simulink model "QuadrangleSimulation"  (R2022b)
settings: Solver=ode4  StartTime=0.0  StopTime=15  FixedStep=ts  MaxStep=0.6  RelTol=1e-3
values from neighbouring files (symbols this model uses):
  N = 20    [QuadrangleMain.m]
  p_left = []    [QuadrangleMain.m]
  p_right = []    [QuadrangleMain.m]
  ra = 0.8    [QuadrangleMain.m]
  rs = 0.5    [QuadrangleMain.m]
  vmax = 3    [QuadrangleMain.m]
settings Model: Creator=51078  LastModifiedBy=51078
settings SolverCC: AlgebraicLoopSolver=TrustRegion
settings DataIOCC: ReturnWorkspaceOutputs=off
settings DebuggingCC: UnconnectedInputMsg=warning  UnconnectedOutputMsg=warning  UnconnectedLineMsg=warning  SFMachineParentedDataDiag=warning  ArithmeticOperatorsInVariantConditions=warning
settings ModelReferenceCC: EnableRefExpFcnMdlSchedulingChecks=on
settings SFSimCC: SimUseLocalCustomCode=off  CustomCodeUndefinedFunction=UseInterfaceOnly
settings RTWCC: RTWUseLocalCustomCode=off  DLArmComputeVersion=19.05
settings CodeAppCC: StateflowObjectComments=on

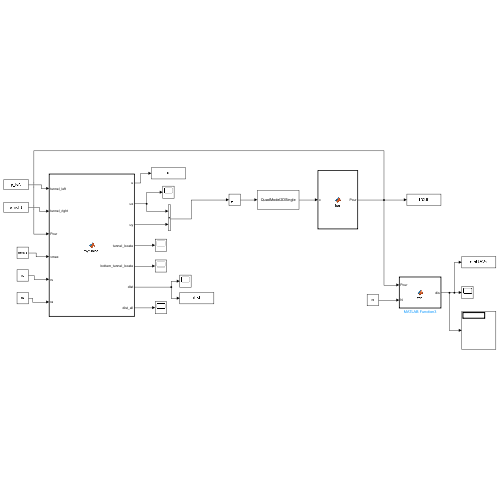
[thumbnail: Simulink's stored preview of the top-level diagram]
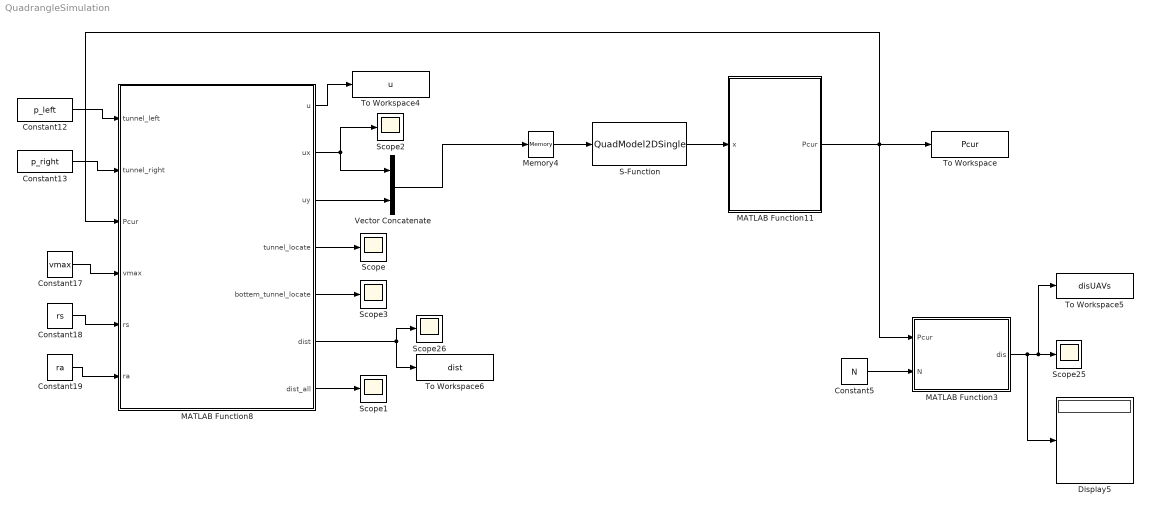
== system QuadrangleSimulation ==
  Constant12 : Constant  Value=p_left
  Constant13 : Constant  Value=p_right
  Constant17 : Constant  Value=vmax
  Constant18 : Constant  Value=rs
  Constant19 : Constant  Value=ra
  Constant5 : Constant  Value=N
  Display5 : Display
  MATLAB Function11 : MATLAB Function  TreatAsAtomicUnit=on
  MATLAB Function3 : MATLAB Function  TreatAsAtomicUnit=on
  MATLAB Function8 : MATLAB Function  TreatAsAtomicUnit=on
  Memory4 : Memory
  S-Function : S-Function  FunctionName=QuadModel2DSingle  SFunctionDeploymentMode=off  EnableBusSupport=off
  Scope{,1..3,25..26} (6 alike) : Scope
  To Workspace : ToWorkspace  VariableName=Pcur  SaveFormat=Timeseries  SampleTime=-1
  To Workspace4 : ToWorkspace  VariableName=u  SaveFormat=Timeseries  SampleTime=-1
  To Workspace5 : ToWorkspace  VariableName=disUAVs  SaveFormat=Timeseries  SampleTime=-1
  To Workspace6 : ToWorkspace  VariableName=dist  SaveFormat=Timeseries  SampleTime=-1
  Vector Concatenate : Concatenate
  wires:
  MATLAB Function8/4(tunnel_locate) -> Scope/1
  Constant12/1 -> MATLAB Function8/1(tunnel_left)
  Constant13/1 -> MATLAB Function8/2(tunnel_right)
  Constant17/1 -> MATLAB Function8/4(vmax)
  Constant18/1 -> MATLAB Function8/5(rs)
  Constant19/1 -> MATLAB Function8/6(ra)
  MATLAB Function11/1(Pcur) -> MATLAB Function8/3(Pcur), To Workspace/1, MATLAB Function3/1(Pcur)
  MATLAB Function3/1(dis) -> Display5/1, To Workspace5/1, Scope25/1
  Constant5/1 -> MATLAB Function3/2(N)
  MATLAB Function8/6(dist) -> Scope26/1, To Workspace6/1
  Memory4/1 -> S-Function/1
  MATLAB Function8/1(u) -> To Workspace4/1
  S-Function/1 -> MATLAB Function11/1(x)
  MATLAB Function8/3(uy) -> Vector Concatenate/2
  MATLAB Function8/2(ux) -> Scope2/1, Vector Concatenate/1
  Vector Concatenate/1 -> Memory4/1
  MATLAB Function8/5(bottem_tunnel_locate) -> Scope3/1
  MATLAB Function8/7(dist_all) -> Scope1/1

== matlab function QuadrangleSimulation/MATLAB Function3 ==
  data: Pcur input; dis output; N input
function dis = fcn(Pcur,N)
dis=10^5;
for i=1:N
    for j=1:N
        if i~=j
            disij=norm(Pcur(i,1:2) - Pcur(j,1:2));
            if disij<dis
                dis=disij;
            end
        end
    end
end

== matlab function QuadrangleSimulation/MATLAB Function8 ==
  data: tunnel_left input; u output size=[N,2]; ux output; uy output; tunnel_right input; Pcur input; vmax input; tunnel_locate output; rs input; ra input; bottem_tunnel_locate output; dist output; dist_all output
function [u,ux,uy,tunnel_locate,bottem_tunnel_locate,dist,dist_all]  = mytunnel(tunnel_left,tunnel_right,Pcur,vmax,rs,ra)
% V21,dis,V31,b_mp,nc,V11,
N=20;

nc=zeros(length(tunnel_left(:,1))-1,2);
nl=zeros(length(tunnel_left(:,1))-1,2);
nr=zeros(length(tunnel_left(:,1))-1,2);
ns=zeros(length(tunnel_left(:,1))-1,2);

c=zeros(length(tunnel_left(:,1))-1,2);
l=zeros(length(tunnel_left(:,1))-1,2);
r=zeros(length(tunnel_left(:,1))-1,2);
s=zeros(length(tunnel_left(:,1))-1,2);


p_fl=zeros(length(tunnel_left(:,1))-1,2);
p_fr=zeros(length(tunnel_left(:,1))-1,2);
p_sl=zeros(length(tunnel_left(:,1))-1,2);
p_sr=zeros(length(tunnel_left(:,1))-1,2);

p_sll=zeros(length(tunnel_left(:,1))-1,2);
p_srr=zeros(length(tunnel_left(:,1))-1,2);

line_left=diff(tunnel_left);
line_right=diff(tunnel_right);
line_end=tunnel_right(2:end,:)-tunnel_left(2:end,:);
line_start=tunnel_right(1:end-1,:)-tunnel_left(1:end-1,:);


for i=1:length(tunnel_left(:,1))-1
    rot_nc=[0 1;-1 0]; %顺时针90度
    rot_nl=[0 1;-1 0];
    rot_nr=[0 -1;1 0]; %逆时针90度
    rot_ns=[0 -1;1 0];
    
    A=rot_nc*line_end(i,:)';
    B=rot_nl*line_left(i,:)';
    C=rot_nr*line_right(i,:)';
    D=rot_ns*line_start(i,:)';
    
    nc(i,:)=(A/norm(A))';
    nl(i,:)=(B/norm(B))';
    nr(i,:)=(C/norm(C))';
    ns(i,:)=(D/norm(D))';
    
    c(i,:)=line_end(i,:)/norm(line_end(i,:));
    l(i,:)=line_left(i,:)/norm(line_left(i,:));
    r(i,:)=line_right(i,:)/norm(line_right(i,:));
    s(i,:)=line_start(i,:)/norm(line_start(i,:));
    
end

for j=1:length(tunnel_left(:,1))-1
    p_fl(j,:)=tunnel_left(j+1,:);
    p_fr(j,:)=tunnel_right(j+1,:);
    p_sl(j,:)=tunnel_left(j,:);
    p_sr(j,:)=tunnel_right(j,:);
    
    p_sll(j,1)=p_sr(j,1)+(l(j,1)*c(j,1)*(p_fl(j,2)-p_sr(j,2))-l(j,2)*c(j,1)*(p_fl(j,1)-p_sr(j,1)))/(l(j,1)*c(j,2)-l(j,2)*c(j,1));
    p_sll(j,2)=p_sr(j,2)+(l(j,1)*c(j,2)*(p_fl(j,2)-p_sr(j,2))-l(j,2)*c(j,2)*(p_fl(j,1)-p_sr(j,1)))/(l(j,1)*c(j,2)-l(j,2)*c(j,1));
    
    p_srr(j,1)=p_sl(j,1)+(r(j,1)*c(j,1)*(p_fr(j,2)-p_sl(j,2))-r(j,2)*c(j,1)*(p_fr(j,1)-p_sl(j,1)))/(r(j,1)*c(j,2)-r(j,2)*c(j,1));
    p_srr(j,2)=p_sl(j,2)+(r(j,1)*c(j,2)*(p_fr(j,2)-p_sl(j,2))-r(j,2)*c(j,2)*(p_fr(j,1)-p_sl(j,1)))/(r(j,1)*c(j,2)-r(j,2)*c(j,1));
end

tunnel_locate=zeros(N,1);
for i=1:N
    for j=1:length(tunnel_left(:,1))-1
        if dot(nl(j,:),(Pcur(i,1:2)-p_fl(j,:)))>=0 && dot(nr(j,:),(Pcur(i,1:2)-p_fr(j,:)))>=0 ...
                && dot(nc(j,:),(Pcur(i,1:2)-p_fr(j,:)))>=0 && dot(ns(j,:),(Pcur(i,1:2)-p_sr(j,:)))>=0
            tunnel_locate(i)=j;
        end
    end
end

e1=zeros(N,2);
V1=zeros(N,2);
V2=zeros(N,2);
V3=zeros(N,2);
V=zeros(N,2);
u=zeros(N,2);
A_mp=zeros(2,2);
b_mp=zeros(2,1);
A_plpr=zeros(2,2);
b_plpr=zeros(2,1);
bottem_tunnel_locate=zeros(N,1);
dist=10^5;
dist_all=zeros(N,1);

rs11=zeros(length(tunnel_left(:,1)),2);
for i=1:length(tunnel_left(:,1))-1
    rs11(i)=rs/min(-dot(nc(i,:),l(i,:)),-dot(nc(i,:),r(i,:)));
end
rs11(length(tunnel_left(:,1)))=rs;
rs1=rs*ones(N,1);
v_line=vmax;

k2=1000;
k3=1000;

for i=1:N
    if tunnel_locate(i)~=0

        p_sll_sr=(p_sll(tunnel_locate(i),:)+p_sr(tunnel_locate(i),:))/2;
        p_srr_sl=(p_srr(tunnel_locate(i),:)+p_sl(tunnel_locate(i),:))/2;
        
        if dot(nl(tunnel_locate(i),:),(p_sll_sr-p_fl(tunnel_locate(i),:)))>=0 && dot(nr(tunnel_locate(i),:),(p_sll_sr-p_fr(tunnel_locate(i),:)))>=0 ...
                && dot(nc(tunnel_locate(i),:),(p_sll_sr-p_fr(tunnel_locate(i),:)))>=0 && dot(ns(tunnel_locate(i),:),(p_sll_sr-p_sr(tunnel_locate(i),:)))>=0
            if dot(nc(tunnel_locate(i),:),(Pcur(i,1:2)-p_sll(tunnel_locate(i),:)))>0
                e1(i,:) = -ns(tunnel_locate(i),:)*(v_line);
                bottem_tunnel_locate(i)=1; %Bottem
                if tunnel_locate(i)==1
                    rs1(i)=rs11(tunnel_locate(i));
                else
                    rs1(i)=max(rs11(tunnel_locate(i)-1),rs11(tunnel_locate(i)));
                end
                
                A_mp(1,1)= 2+l(tunnel_locate(i),2)*s(tunnel_locate(i),1)/(l(tunnel_locate(i),1)*s(tunnel_locate(i),2)-l(tunnel_locate(i),2)*s(tunnel_locate(i),1))+r(tunnel_locate(i),2)*s(tunnel_locate(i),1)/(r(tunnel_locate(i),1)*s(tunnel_locate(i),2)-r(tunnel_locate(i),2)*s(tunnel_locate(i),1));
                A_mp(1,2)=  -l(tunnel_locate(i),1)*s(tunnel_locate(i),1)/(l(tunnel_locate(i),1)*s(tunnel_locate(i),2)-l(tunnel_locate(i),2)*s(tunnel_locate(i),1))-r(tunnel_locate(i),1)*s(tunnel_locate(i),1)/(r(tunnel_locate(i),1)*s(tunnel_locate(i),2)-r(tunnel_locate(i),2)*s(tunnel_locate(i),1));
                A_mp(2,1)=   l(tunnel_locate(i),2)*s(tunnel_locate(i),2)/(l(tunnel_locate(i),1)*s(tunnel_locate(i),2)-l(tunnel_locate(i),2)*s(tunnel_locate(i),1))+r(tunnel_locate(i),2)*s(tunnel_locate(i),2)/(r(tunnel_locate(i),1)*s(tunnel_locate(i),2)-r(tunnel_locate(i),2)*s(tunnel_locate(i),1));
                A_mp(2,2)= 2-l(tunnel_locate(i),1)*s(tunnel_locate(i),2)/(l(tunnel_locate(i),1)*s(tunnel_locate(i),2)-l(tunnel_locate(i),2)*s(tunnel_locate(i),1))-r(tunnel_locate(i),1)*s(tunnel_locate(i),2)/(r(tunnel_locate(i),1)*s(tunnel_locate(i),2)-r(tunnel_locate(i),2)*s(tunnel_locate(i),1));
                A_mp=A_mp/2;
                
                b_mp(1,1)=  (l(tunnel_locate(i),1)*s(tunnel_locate(i),1)*p_fl(tunnel_locate(i),2)-l(tunnel_locate(i),2)*s(tunnel_locate(i),1)*p_fl(tunnel_locate(i),1))/(l(tunnel_locate(i),1)*s(tunnel_locate(i),2)-l(tunnel_locate(i),2)*s(tunnel_locate(i),1))+(r(tunnel_locate(i),1)*s(tunnel_locate(i),1)*p_fr(tunnel_locate(i),2)-r(tunnel_locate(i),2)*s(tunnel_locate(i),1)*p_fr(tunnel_locate(i),1))/(r(tunnel_locate(i),1)*s(tunnel_locate(i),2)-r(tunnel_locate(i),2)*s(tunnel_locate(i),1));
                b_mp(2,1)=  (l(tunnel_locate(i),1)*s(tunnel_locate(i),2)*p_fl(tunnel_locate(i),2)-l(tunnel_locate(i),2)*s(tunnel_locate(i),2)*p_fl(tunnel_locate(i),1))/(l(tunnel_locate(i),1)*s(tunnel_locate(i),2)-l(tunnel_locate(i),2)*s(tunnel_locate(i),1))+(r(tunnel_locate(i),1)*s(tunnel_locate(i),2)*p_fr(tunnel_locate(i),2)-r(tunnel_locate(i),2)*s(tunnel_locate(i),2)*p_fr(tunnel_locate(i),1))/(r(tunnel_locate(i),1)*s(tunnel_locate(i),2)-r(tunnel_locate(i),2)*s(tunnel_locate(i),1));
                b_mp=b_mp/2;
                                
                A_plpr(1,1)= l(tunnel_locate(i),2)*s(tunnel_locate(i),1)/(l(tunnel_locate(i),1)*s(tunnel_locate(i),2)-l(tunnel_locate(i),2)*s(tunnel_locate(i),1))-r(tunnel_locate(i),2)*s(tunnel_locate(i),1)/(r(tunnel_locate(i),1)*s(tunnel_locate(i),2)-r(tunnel_locate(i),2)*s(tunnel_locate(i),1));
                A_plpr(1,2)=-l(tunnel_locate(i),1)*s(tunnel_locate(i),1)/(l(tunnel_locate(i),1)*s(tunnel_locate(i),2)-l(tunnel_locate(i),2)*s(tunnel_locate(i),1))+r(tunnel_locate(i),1)*s(tunnel_locate(i),1)/(r(tunnel_locate(i),1)*s(tunnel_locate(i),2)-r(tunnel_locate(i),2)*s(tunnel_locate(i),1));
                A_plpr(2,1)= l(tunnel_locate(i),2)*s(tunnel_locate(i),2)/(l(tunnel_locate(i),1)*s(tunnel_locate(i),2)-l(tunnel_locate(i),2)*s(tunnel_locate(i),1))-r(tunnel_locate(i),2)*s(tunnel_locate(i),2)/(r(tunnel_locate(i),1)*s(tunnel_locate(i),2)-r(tunnel_locate(i),2)*s(tunnel_locate(i),1));
                A_plpr(2,2)=-l(tunnel_locate(i),1)*s(tunnel_locate(i),2)/(l(tunnel_locate(i),1)*s(tunnel_locate(i),2)-l(tunnel_locate(i),2)*s(tunnel_locate(i),1))+r(tunnel_locate(i),1)*s(tunnel_locate(i),2)/(r(tunnel_locate(i),1)*s(tunnel_locate(i),2)-r(tunnel_locate(i),2)*s(tunnel_locate(i),1));
                
                b_plpr(1,1)=(l(tunnel_locate(i),1)*s(tunnel_locate(i),1)*p_fl(tunnel_locate(i),2)-l(tunnel_locate(i),2)*s(tunnel_locate(i),1)*p_fl(tunnel_locate(i),1))/(l(tunnel_locate(i),1)*s(tunnel_locate(i),2)-l(tunnel_locate(i),2)*s(tunnel_locate(i),1))-(r(tunnel_locate(i),1)*s(tunnel_locate(i),1)*p_fr(tunnel_locate(i),2)-r(tunnel_locate(i),2)*s(tunnel_locate(i),1)*p_fr(tunnel_locate(i),1))/(r(tunnel_locate(i),1)*s(tunnel_locate(i),2)-r(tunnel_locate(i),2)*s(tunnel_locate(i),1));
                b_plpr(2,1)=(l(tunnel_locate(i),1)*s(tunnel_locate(i),2)*p_fl(tunnel_locate(i),2)-l(tunnel_locate(i),2)*s(tunnel_locate(i),2)*p_fl(tunnel_locate(i),1))/(l(tunnel_locate(i),1)*s(tunnel_locate(i),2)-l(tunnel_locate(i),2)*s(tunnel_locate(i),1))-(r(tunnel_locate(i),1)*s(tunnel_locate(i),2)*p_fr(tunnel_locate(i),2)-r(tunnel_locate(i),2)*s(tunnel_locate(i),2)*p_fr(tunnel_locate(i),1))/(r(tunnel_locate(i),1)*s(tunnel_locate(i),2)-r(tunnel_locate(i),2)*s(tunnel_locate(i),1));
            elseif dot(nc(tunnel_locate(i),:),(Pcur(i,1:2)-p_sll(tunnel_locate(i),:)))<=0
                e1(i,:) = nc(tunnel_locate(i),:)*(v_line);
                rs1(i)=max(rs11(tunnel_locate(i)),rs11(tunnel_locate(i)+1));
                bottem_tunnel_locate(i)=9; %Inscribe
                
                A_mp(1,1)= 2+l(tunnel_locate(i),2)*c(tunnel_locate(i),1)/(l(tunnel_locate(i),1)*c(tunnel_locate(i),2)-l(tunnel_locate(i),2)*c(tunnel_locate(i),1))+r(tunnel_locate(i),2)*c(tunnel_locate(i),1)/(r(tunnel_locate(i),1)*c(tunnel_locate(i),2)-r(tunnel_locate(i),2)*c(tunnel_locate(i),1));
                A_mp(1,2)=  -l(tunnel_locate(i),1)*c(tunnel_locate(i),1)/(l(tunnel_locate(i),1)*c(tunnel_locate(i),2)-l(tunnel_locate(i),2)*c(tunnel_locate(i),1))-r(tunnel_locate(i),1)*c(tunnel_locate(i),1)/(r(tunnel_locate(i),1)*c(tunnel_locate(i),2)-r(tunnel_locate(i),2)*c(tunnel_locate(i),1));
                A_mp(2,1)=   l(tunnel_locate(i),2)*c(tunnel_locate(i),2)/(l(tunnel_locate(i),1)*c(tunnel_locate(i),2)-l(tunnel_locate(i),2)*c(tunnel_locate(i),1))+r(tunnel_locate(i),2)*c(tunnel_locate(i),2)/(r(tunnel_locate(i),1)*c(tunnel_locate(i),2)-r(tunnel_locate(i),2)*c(tunnel_locate(i),1));
                A_mp(2,2)= 2-l(tunnel_locate(i),1)*c(tunnel_locate(i),2)/(l(tunnel_locate(i),1)*c(tunnel_locate(i),2)-l(tunnel_locate(i),2)*c(tunnel_locate(i),1))-r(tunnel_locate(i),1)*c(tunnel_locate(i),2)/(r(tunnel_locate(i),1)*c(tunnel_locate(i),2)-r(tunnel_locate(i),2)*c(tunnel_locate(i),1));
                A_mp=A_mp/2;
                
                b_mp(1,1)=  (l(tunnel_locate(i),1)*c(tunnel_locate(i),1)*p_fl(tunnel_locate(i),2)-l(tunnel_locate(i),2)*c(tunnel_locate(i),1)*p_fl(tunnel_locate(i),1))/(l(tunnel_locate(i),1)*c(tunnel_locate(i),2)-l(tunnel_locate(i),2)*c(tunnel_locate(i),1))+(r(tunnel_locate(i),1)*c(tunnel_locate(i),1)*p_fr(tunnel_locate(i),2)-r(tunnel_locate(i),2)*c(tunnel_locate(i),1)*p_fr(tunnel_locate(i),1))/(r(tunnel_locate(i),1)*c(tunnel_locate(i),2)-r(tunnel_locate(i),2)*c(tunnel_locate(i),1));
                b_mp(2,1)=  (l(tunnel_locate(i),1)*c(tunnel_locate(i),2)*p_fl(tunnel_locate(i),2)-l(tunnel_locate(i),2)*c(tunnel_locate(i),2)*p_fl(tunnel_locate(i),1))/(l(tunnel_locate(i),1)*c(tunnel_locate(i),2)-l(tunnel_locate(i),2)*c(tunnel_locate(i),1))+(r(tunnel_locate(i),1)*c(tunnel_locate(i),2)*p_fr(tunnel_locate(i),2)-r(tunnel_locate(i),2)*c(tunnel_locate(i),2)*p_fr(tunnel_locate(i),1))/(r(tunnel_locate(i),1)*c(tunnel_locate(i),2)-r(tunnel_locate(i),2)*c(tunnel_locate(i),1));
                b_mp=b_mp/2;
                               
                A_plpr(1,1)= l(tunnel_locate(i),2)*c(tunnel_locate(i),1)/(l(tunnel_locate(i),1)*c(tunnel_locate(i),2)-l(tunnel_locate(i),2)*c(tunnel_locate(i),1))-r(tunnel_locate(i),2)*c(tunnel_locate(i),1)/(r(tunnel_locate(i),1)*c(tunnel_locate(i),2)-r(tunnel_locate(i),2)*c(tunnel_locate(i),1));
                A_plpr(1,2)=-l(tunnel_locate(i),1)*c(tunnel_locate(i),1)/(l(tunnel_locate(i),1)*c(tunnel_locate(i),2)-l(tunnel_locate(i),2)*c(tunnel_locate(i),1))+r(tunnel_locate(i),1)*c(tunnel_locate(i),1)/(r(tunnel_locate(i),1)*c(tunnel_locate(i),2)-r(tunnel_locate(i),2)*c(tunnel_locate(i),1));
                A_plpr(2,1)= l(tunnel_locate(i),2)*c(tunnel_locate(i),2)/(l(tunnel_locate(i),1)*c(tunnel_locate(i),2)-l(tunnel_locate(i),2)*c(tunnel_locate(i),1))-r(tunnel_locate(i),2)*c(tunnel_locate(i),2)/(r(tunnel_locate(i),1)*c(tunnel_locate(i),2)-r(tunnel_locate(i),2)*c(tunnel_locate(i),1));
                A_plpr(2,2)=-l(tunnel_locate(i),1)*c(tunnel_locate(i),2)/(l(tunnel_locate(i),1)*c(tunnel_locate(i),2)-l(tunnel_locate(i),2)*c(tunnel_locate(i),1))+r(tunnel_locate(i),1)*c(tunnel_locate(i),2)/(r(tunnel_locate(i),1)*c(tunnel_locate(i),2)-r(tunnel_locate(i),2)*c(tunnel_locate(i),1));
                
                b_plpr(1,1)=(l(tunnel_locate(i),1)*c(tunnel_locate(i),1)*p_fl(tunnel_locate(i),2)-l(tunnel_locate(i),2)*c(tunnel_locate(i),1)*p_fl(tunnel_locate(i),1))/(l(tunnel_locate(i),1)*c(tunnel_locate(i),2)-l(tunnel_locate(i),2)*c(tunnel_locate(i),1))-(r(tunnel_locate(i),1)*c(tunnel_locate(i),1)*p_fr(tunnel_locate(i),2)-r(tunnel_locate(i),2)*c(tunnel_locate(i),1)*p_fr(tunnel_locate(i),1))/(r(tunnel_locate(i),1)*c(tunnel_locate(i),2)-r(tunnel_locate(i),2)*c(tunnel_locate(i),1));
                b_plpr(2,1)=(l(tunnel_locate(i),1)*c(tunnel_locate(i),2)*p_fl(tunnel_locate(i),2)-l(tunnel_locate(i),2)*c(tunnel_locate(i),2)*p_fl(tunnel_locate(i),1))/(l(tunnel_locate(i),1)*c(tunnel_locate(i),2)-l(tunnel_locate(i),2)*c(tunnel_locate(i),1))-(r(tunnel_locate(i),1)*c(tunnel_locate(i),2)*p_fr(tunnel_locate(i),2)-r(tunnel_locate(i),2)*c(tunnel_locate(i),2)*p_fr(tunnel_locate(i),1))/(r(tunnel_locate(i),1)*c(tunnel_locate(i),2)-r(tunnel_locate(i),2)*c(tunnel_locate(i),1));
            end
        elseif dot(nl(tunnel_locate(i),:),(p_srr_sl-p_fl(tunnel_locate(i),:)))>=0 && dot(nr(tunnel_locate(i),:),(p_srr_sl-p_fr(tunnel_locate(i),:)))>=0 ...
                && dot(nc(tunnel_locate(i),:),(p_srr_sl-p_fr(tunnel_locate(i),:)))>=0 && dot(ns(tunnel_locate(i),:),(p_srr_sl-p_sr(tunnel_locate(i),:)))>=0
            if dot(nc(tunnel_locate(i),:),(Pcur(i,1:2)-p_srr(tunnel_locate(i),:)))>0
                e1(i,:) = -ns(tunnel_locate(i),:)*(v_line); %Bottem
                bottem_tunnel_locate(i)=2;
                if tunnel_locate(i)==1
                    rs1(i)=rs11(tunnel_locate(i));
                else
                    rs1(i)=max(rs11(tunnel_locate(i)-1),rs11(tunnel_locate(i)));
                end
                
                A_mp(1,1)= 2+l(tunnel_locate(i),2)*s(tunnel_locate(i),1)/(l(tunnel_locate(i),1)*s(tunnel_locate(i),2)-l(tunnel_locate(i),2)*s(tunnel_locate(i),1))+r(tunnel_locate(i),2)*s(tunnel_locate(i),1)/(r(tunnel_locate(i),1)*s(tunnel_locate(i),2)-r(tunnel_locate(i),2)*s(tunnel_locate(i),1));
                A_mp(1,2)=  -l(tunnel_locate(i),1)*s(tunnel_locate(i),1)/(l(tunnel_locate(i),1)*s(tunnel_locate(i),2)-l(tunnel_locate(i),2)*s(tunnel_locate(i),1))-r(tunnel_locate(i),1)*s(tunnel_locate(i),1)/(r(tunnel_locate(i),1)*s(tunnel_locate(i),2)-r(tunnel_locate(i),2)*s(tunnel_locate(i),1));
                A_mp(2,1)=   l(tunnel_locate(i),2)*s(tunnel_locate(i),2)/(l(tunnel_locate(i),1)*s(tunnel_locate(i),2)-l(tunnel_locate(i),2)*s(tunnel_locate(i),1))+r(tunnel_locate(i),2)*s(tunnel_locate(i),2)/(r(tunnel_locate(i),1)*s(tunnel_locate(i),2)-r(tunnel_locate(i),2)*s(tunnel_locate(i),1));
                A_mp(2,2)= 2-l(tunnel_locate(i),1)*s(tunnel_locate(i),2)/(l(tunnel_locate(i),1)*s(tunnel_locate(i),2)-l(tunnel_locate(i),2)*s(tunnel_locate(i),1))-r(tunnel_locate(i),1)*s(tunnel_locate(i),2)/(r(tunnel_locate(i),1)*s(tunnel_locate(i),2)-r(tunnel_locate(i),2)*s(tunnel_locate(i),1));
                A_mp=A_mp/2;
                
                b_mp(1,1)=  (l(tunnel_locate(i),1)*s(tunnel_locate(i),1)*p_fl(tunnel_locate(i),2)-l(tunnel_locate(i),2)*s(tunnel_locate(i),1)*p_fl(tunnel_locate(i),1))/(l(tunnel_locate(i),1)*s(tunnel_locate(i),2)-l(tunnel_locate(i),2)*s(tunnel_locate(i),1))+(r(tunnel_locate(i),1)*s(tunnel_locate(i),1)*p_fr(tunnel_locate(i),2)-r(tunnel_locate(i),2)*s(tunnel_locate(i),1)*p_fr(tunnel_locate(i),1))/(r(tunnel_locate(i),1)*s(tunnel_locate(i),2)-r(tunnel_locate(i),2)*s(tunnel_locate(i),1));
                b_mp(2,1)=  (l(tunnel_locate(i),1)*s(tunnel_locate(i),2)*p_fl(tunnel_locate(i),2)-l(tunnel_locate(i),2)*s(tunnel_locate(i),2)*p_fl(tunnel_locate(i),1))/(l(tunnel_locate(i),1)*s(tunnel_locate(i),2)-l(tunnel_locate(i),2)*s(tunnel_locate(i),1))+(r(tunnel_locate(i),1)*s(tunnel_locate(i),2)*p_fr(tunnel_locate(i),2)-r(tunnel_locate(i),2)*s(tunnel_locate(i),2)*p_fr(tunnel_locate(i),1))/(r(tunnel_locate(i),1)*s(tunnel_locate(i),2)-r(tunnel_locate(i),2)*s(tunnel_locate(i),1));
                b_mp=b_mp/2;
                
                A_plpr(1,1)= l(tunnel_locate(i),2)*s(tunnel_locate(i),1)/(l(tunnel_locate(i),1)*s(tunnel_locate(i),2)-l(tunnel_locate(i),2)*s(tunnel_locate(i),1))-r(tunnel_locate(i),2)*s(tunnel_locate(i),1)/(r(tunnel_locate(i),1)*s(tunnel_locate(i),2)-r(tunnel_locate(i),2)*s(tunnel_locate(i),1));
                A_plpr(1,2)=-l(tunnel_locate(i),1)*s(tunnel_locate(i),1)/(l(tunnel_locate(i),1)*s(tunnel_locate(i),2)-l(tunnel_locate(i),2)*s(tunnel_locate(i),1))+r(tunnel_locate(i),1)*s(tunnel_locate(i),1)/(r(tunnel_locate(i),1)*s(tunnel_locate(i),2)-r(tunnel_locate(i),2)*s(tunnel_locate(i),1));
                A_plpr(2,1)= l(tunnel_locate(i),2)*s(tunnel_locate(i),2)/(l(tunnel_locate(i),1)*s(tunnel_locate(i),2)-l(tunnel_locate(i),2)*s(tunnel_locate(i),1))-r(tunnel_locate(i),2)*s(tunnel_locate(i),2)/(r(tunnel_locate(i),1)*s(tunnel_locate(i),2)-r(tunnel_locate(i),2)*s(tunnel_locate(i),1));
                A_plpr(2,2)=-l(tunnel_locate(i),1)*s(tunnel_locate(i),2)/(l(tunnel_locate(i),1)*s(tunnel_locate(i),2)-l(tunnel_locate(i),2)*s(tunnel_locate(i),1))+r(tunnel_locate(i),1)*s(tunnel_locate(i),2)/(r(tunnel_locate(i),1)*s(tunnel_locate(i),2)-r(tunnel_locate(i),2)*s(tunnel_locate(i),1));
                
                b_plpr(1,1)=(l(tunnel_locate(i),1)*s(tunnel_locate(i),1)*p_fl(tunnel_locate(i),2)-l(tunnel_locate(i),2)*s(tunnel_locate(i),1)*p_fl(tunnel_locate(i),1))/(l(tunnel_locate(i),1)*s(tunnel_locate(i),2)-l(tunnel_locate(i),2)*s(tunnel_locate(i),1))-(r(tunnel_locate(i),1)*s(tunnel_locate(i),1)*p_fr(tunnel_locate(i),2)-r(tunnel_locate(i),2)*s(tunnel_locate(i),1)*p_fr(tunnel_locate(i),1))/(r(tunnel_locate(i),1)*s(tunnel_locate(i),2)-r(tunnel_locate(i),2)*s(tunnel_locate(i),1));
                b_plpr(2,1)=(l(tunnel_locate(i),1)*s(tunnel_locate(i),2)*p_fl(tunnel_locate(i),2)-l(tunnel_locate(i),2)*s(tunnel_locate(i),2)*p_fl(tunnel_locate(i),1))/(l(tunnel_locate(i),1)*s(tunnel_locate(i),2)-l(tunnel_locate(i),2)*s(tunnel_locate(i),1))-(r(tunnel_locate(i),1)*s(tunnel_locate(i),2)*p_fr(tunnel_locate(i),2)-r(tunnel_locate(i),2)*s(tunnel_locate(i),2)*p_fr(tunnel_locate(i),1))/(r(tunnel_locate(i),1)*s(tunnel_locate(i),2)-r(tunnel_locate(i),2)*s(tunnel_locate(i),1));            
            elseif dot(nc(tunnel_locate(i),:),(Pcur(i,1:2)-p_srr(tunnel_locate(i),:)))<=0
                e1(i,:) = nc(tunnel_locate(i),:)*(v_line);
                rs1(i)=max(rs11(tunnel_locate(i)),rs11(tunnel_locate(i)+1));
                bottem_tunnel_locate(i)=10; %Inscribe
                
                A_mp(1,1)= 2+l(tunnel_locate(i),2)*c(tunnel_locate(i),1)/(l(tunnel_locate(i),1)*c(tunnel_locate(i),2)-l(tunnel_locate(i),2)*c(tunnel_locate(i),1))+r(tunnel_locate(i),2)*c(tunnel_locate(i),1)/(r(tunnel_locate(i),1)*c(tunnel_locate(i),2)-r(tunnel_locate(i),2)*c(tunnel_locate(i),1));
                A_mp(1,2)=  -l(tunnel_locate(i),1)*c(tunnel_locate(i),1)/(l(tunnel_locate(i),1)*c(tunnel_locate(i),2)-l(tunnel_locate(i),2)*c(tunnel_locate(i),1))-r(tunnel_locate(i),1)*c(tunnel_locate(i),1)/(r(tunnel_locate(i),1)*c(tunnel_locate(i),2)-r(tunnel_locate(i),2)*c(tunnel_locate(i),1));
                A_mp(2,1)=   l(tunnel_locate(i),2)*c(tunnel_locate(i),2)/(l(tunnel_locate(i),1)*c(tunnel_locate(i),2)-l(tunnel_locate(i),2)*c(tunnel_locate(i),1))+r(tunnel_locate(i),2)*c(tunnel_locate(i),2)/(r(tunnel_locate(i),1)*c(tunnel_locate(i),2)-r(tunnel_locate(i),2)*c(tunnel_locate(i),1));
                A_mp(2,2)= 2-l(tunnel_locate(i),1)*c(tunnel_locate(i),2)/(l(tunnel_locate(i),1)*c(tunnel_locate(i),2)-l(tunnel_locate(i),2)*c(tunnel_locate(i),1))-r(tunnel_locate(i),1)*c(tunnel_locate(i),2)/(r(tunnel_locate(i),1)*c(tunnel_locate(i),2)-r(tunnel_locate(i),2)*c(tunnel_locate(i),1));
                A_mp=A_mp/2;
                
                b_mp(1,1)=  (l(tunnel_locate(i),1)*c(tunnel_locate(i),1)*p_fl(tunnel_locate(i),2)-l(tunnel_locate(i),2)*c(tunnel_locate(i),1)*p_fl(tunnel_locate(i),1))/(l(tunnel_locate(i),1)*c(tunnel_locate(i),2)-l(tunnel_locate(i),2)*c(tunnel_locate(i),1))+(r(tunnel_locate(i),1)*c(tunnel_locate(i),1)*p_fr(tunnel_locate(i),2)-r(tunnel_locate(i),2)*c(tunnel_locate(i),1)*p_fr(tunnel_locate(i),1))/(r(tunnel_locate(i),1)*c(tunnel_locate(i),2)-r(tunnel_locate(i),2)*c(tunnel_locate(i),1));
                b_mp(2,1)=  (l(tunnel_locate(i),1)*c(tunnel_locate(i),2)*p_fl(tunnel_locate(i),2)-l(tunnel_locate(i),2)*c(tunnel_locate(i),2)*p_fl(tunnel_locate(i),1))/(l(tunnel_locate(i),1)*c(tunnel_locate(i),2)-l(tunnel_locate(i),2)*c(tunnel_locate(i),1))+(r(tunnel_locate(i),1)*c(tunnel_locate(i),2)*p_fr(tunnel_locate(i),2)-r(tunnel_locate(i),2)*c(tunnel_locate(i),2)*p_fr(tunnel_locate(i),1))/(r(tunnel_locate(i),1)*c(tunnel_locate(i),2)-r(tunnel_locate(i),2)*c(tunnel_locate(i),1));
                b_mp=b_mp/2;
                
                A_plpr(1,1)= l(tunnel_locate(i),2)*c(tunnel_locate(i),1)/(l(tunnel_locate(i),1)*c(tunnel_locate(i),2)-l(tunnel_locate(i),2)*c(tunnel_locate(i),1))-r(tunnel_locate(i),2)*c(tunnel_locate(i),1)/(r(tunnel_locate(i),1)*c(tunnel_locate(i),2)-r(tunnel_locate(i),2)*c(tunnel_locate(i),1));
                A_plpr(1,2)=-l(tunnel_locate(i),1)*c(tunnel_locate(i),1)/(l(tunnel_locate(i),1)*c(tunnel_locate(i),2)-l(tunnel_locate(i),2)*c(tunnel_locate(i),1))+r(tunnel_locate(i),1)*c(tunnel_locate(i),1)/(r(tunnel_locate(i),1)*c(tunnel_locate(i),2)-r(tunnel_locate(i),2)*c(tunnel_locate(i),1));
                A_plpr(2,1)= l(tunnel_locate(i),2)*c(tunnel_locate(i),2)/(l(tunnel_locate(i),1)*c(tunnel_locate(i),2)-l(tunnel_locate(i),2)*c(tunnel_locate(i),1))-r(tunnel_locate(i),2)*c(tunnel_locate(i),2)/(r(tunnel_locate(i),1)*c(tunnel_locate(i),2)-r(tunnel_locate(i),2)*c(tunnel_locate(i),1));
                A_plpr(2,2)=-l(tunnel_locate(i),1)*c(tunnel_locate(i),2)/(l(tunnel_locate(i),1)*c(tunnel_locate(i),2)-l(tunnel_locate(i),2)*c(tunnel_locate(i),1))+r(tunnel_locate(i),1)*c(tunnel_locate(i),2)/(r(tunnel_locate(i),1)*c(tunnel_locate(i),2)-r(tunnel_locate(i),2)*c(tunnel_locate(i),1));
                
                b_plpr(1,1)=(l(tunnel_locate(i),1)*c(tunnel_locate(i),1)*p_fl(tunnel_locate(i),2)-l(tunnel_locate(i),2)*c(tunnel_locate(i),1)*p_fl(tunnel_locate(i),1))/(l(tunnel_locate(i),1)*c(tunnel_locate(i),2)-l(tunnel_locate(i),2)*c(tunnel_locate(i),1))-(r(tunnel_locate(i),1)*c(tunnel_locate(i),1)*p_fr(tunnel_locate(i),2)-r(tunnel_locate(i),2)*c(tunnel_locate(i),1)*p_fr(tunnel_locate(i),1))/(r(tunnel_locate(i),1)*c(tunnel_locate(i),2)-r(tunnel_locate(i),2)*c(tunnel_locate(i),1));
                b_plpr(2,1)=(l(tunnel_locate(i),1)*c(tunnel_locate(i),2)*p_fl(tunnel_locate(i),2)-l(tunnel_locate(i),2)*c(tunnel_locate(i),2)*p_fl(tunnel_locate(i),1))/(l(tunnel_locate(i),1)*c(tunnel_locate(i),2)-l(tunnel_locate(i),2)*c(tunnel_locate(i),1))-(r(tunnel_locate(i),1)*c(tunnel_locate(i),2)*p_fr(tunnel_locate(i),2)-r(tunnel_locate(i),2)*c(tunnel_locate(i),2)*p_fr(tunnel_locate(i),1))/(r(tunnel_locate(i),1)*c(tunnel_locate(i),2)-r(tunnel_locate(i),2)*c(tunnel_locate(i),1));
            end
        else
            e1(i,:) = nc(tunnel_locate(i),:)*(v_line);
            rs1(i)=max(rs11(tunnel_locate(i)),rs11(tunnel_locate(i)+1));
            bottem_tunnel_locate(i)=3; %TiXing
            A_mp(1,1)= 2+l(tunnel_locate(i),2)*c(tunnel_locate(i),1)/(l(tunnel_locate(i),1)*c(tunnel_locate(i),2)-l(tunnel_locate(i),2)*c(tunnel_locate(i),1))+r(tunnel_locate(i),2)*c(tunnel_locate(i),1)/(r(tunnel_locate(i),1)*c(tunnel_locate(i),2)-r(tunnel_locate(i),2)*c(tunnel_locate(i),1));
            A_mp(1,2)=  -l(tunnel_locate(i),1)*c(tunnel_locate(i),1)/(l(tunnel_locate(i),1)*c(tunnel_locate(i),2)-l(tunnel_locate(i),2)*c(tunnel_locate(i),1))-r(tunnel_locate(i),1)*c(tunnel_locate(i),1)/(r(tunnel_locate(i),1)*c(tunnel_locate(i),2)-r(tunnel_locate(i),2)*c(tunnel_locate(i),1));
            A_mp(2,1)=   l(tunnel_locate(i),2)*c(tunnel_locate(i),2)/(l(tunnel_locate(i),1)*c(tunnel_locate(i),2)-l(tunnel_locate(i),2)*c(tunnel_locate(i),1))+r(tunnel_locate(i),2)*c(tunnel_locate(i),2)/(r(tunnel_locate(i),1)*c(tunnel_locate(i),2)-r(tunnel_locate(i),2)*c(tunnel_locate(i),1));
            A_mp(2,2)= 2-l(tunnel_locate(i),1)*c(tunnel_locate(i),2)/(l(tunnel_locate(i),1)*c(tunnel_locate(i),2)-l(tunnel_locate(i),2)*c(tunnel_locate(i),1))-r(tunnel_locate(i),1)*c(tunnel_locate(i),2)/(r(tunnel_locate(i),1)*c(tunnel_locate(i),2)-r(tunnel_locate(i),2)*c(tunnel_locate(i),1));
            A_mp=A_mp/2;
            
            b_mp(1,1)=  (l(tunnel_locate(i),1)*c(tunnel_locate(i),1)*p_fl(tunnel_locate(i),2)-l(tunnel_locate(i),2)*c(tunnel_locate(i),1)*p_fl(tunnel_locate(i),1))/(l(tunnel_locate(i),1)*c(tunnel_locate(i),2)-l(tunnel_locate(i),2)*c(tunnel_locate(i),1))+(r(tunnel_locate(i),1)*c(tunnel_locate(i),1)*p_fr(tunnel_locate(i),2)-r(tunnel_locate(i),2)*c(tunnel_locate(i),1)*p_fr(tunnel_locate(i),1))/(r(tunnel_locate(i),1)*c(tunnel_locate(i),2)-r(tunnel_locate(i),2)*c(tunnel_locate(i),1));
            b_mp(2,1)=  (l(tunnel_locate(i),1)*c(tunnel_locate(i),2)*p_fl(tunnel_locate(i),2)-l(tunnel_locate(i),2)*c(tunnel_locate(i),2)*p_fl(tunnel_locate(i),1))/(l(tunnel_locate(i),1)*c(tunnel_locate(i),2)-l(tunnel_locate(i),2)*c(tunnel_locate(i),1))+(r(tunnel_locate(i),1)*c(tunnel_locate(i),2)*p_fr(tunnel_locate(i),2)-r(tunnel_locate(i),2)*c(tunnel_locate(i),2)*p_fr(tunnel_locate(i),1))/(r(tunnel_locate(i),1)*c(tunnel_locate(i),2)-r(tunnel_locate(i),2)*c(tunnel_locate(i),1));
            b_mp=b_mp/2;
            
            A_plpr(1,1)= l(tunnel_locate(i),2)*c(tunnel_locate(i),1)/(l(tunnel_locate(i),1)*c(tunnel_locate(i),2)-l(tunnel_locate(i),2)*c(tunnel_locate(i),1))-r(tunnel_locate(i),2)*c(tunnel_locate(i),1)/(r(tunnel_locate(i),1)*c(tunnel_locate(i),2)-r(tunnel_locate(i),2)*c(tunnel_locate(i),1));
            A_plpr(1,2)=-l(tunnel_locate(i),1)*c(tunnel_locate(i),1)/(l(tunnel_locate(i),1)*c(tunnel_locate(i),2)-l(tunnel_locate(i),2)*c(tunnel_locate(i),1))+r(tunnel_locate(i),1)*c(tunnel_locate(i),1)/(r(tunnel_locate(i),1)*c(tunnel_locate(i),2)-r(tunnel_locate(i),2)*c(tunnel_locate(i),1));
            A_plpr(2,1)= l(tunnel_locate(i),2)*c(tunnel_locate(i),2)/(l(tunnel_locate(i),1)*c(tunnel_locate(i),2)-l(tunnel_locate(i),2)*c(tunnel_locate(i),1))-r(tunnel_locate(i),2)*c(tunnel_locate(i),2)/(r(tunnel_locate(i),1)*c(tunnel_locate(i),2)-r(tunnel_locate(i),2)*c(tunnel_locate(i),1));
            A_plpr(2,2)=-l(tunnel_locate(i),1)*c(tunnel_locate(i),2)/(l(tunnel_locate(i),1)*c(tunnel_locate(i),2)-l(tunnel_locate(i),2)*c(tunnel_locate(i),1))+r(tunnel_locate(i),1)*c(tunnel_locate(i),2)/(r(tunnel_locate(i),1)*c(tunnel_locate(i),2)-r(tunnel_locate(i),2)*c(tunnel_locate(i),1));
            
            b_plpr(1,1)=(l(tunnel_locate(i),1)*c(tunnel_locate(i),1)*p_fl(tunnel_locate(i),2)-l(tunnel_locate(i),2)*c(tunnel_locate(i),1)*p_fl(tunnel_locate(i),1))/(l(tunnel_locate(i),1)*c(tunnel_locate(i),2)-l(tunnel_locate(i),2)*c(tunnel_locate(i),1))-(r(tunnel_locate(i),1)*c(tunnel_locate(i),1)*p_fr(tunnel_locate(i),2)-r(tunnel_locate(i),2)*c(tunnel_locate(i),1)*p_fr(tunnel_locate(i),1))/(r(tunnel_locate(i),1)*c(tunnel_locate(i),2)-r(tunnel_locate(i),2)*c(tunnel_locate(i),1));
            b_plpr(2,1)=(l(tunnel_locate(i),1)*c(tunnel_locate(i),2)*p_fl(tunnel_locate(i),2)-l(tunnel_locate(i),2)*c(tunnel_locate(i),2)*p_fl(tunnel_locate(i),1))/(l(tunnel_locate(i),1)*c(tunnel_locate(i),2)-l(tunnel_locate(i),2)*c(tunnel_locate(i),1))-(r(tunnel_locate(i),1)*c(tunnel_locate(i),2)*p_fr(tunnel_locate(i),2)-r(tunnel_locate(i),2)*c(tunnel_locate(i),2)*p_fr(tunnel_locate(i),1))/(r(tunnel_locate(i),1)*c(tunnel_locate(i),2)-r(tunnel_locate(i),2)*c(tunnel_locate(i),1));           
        end
        
        
        if i>=1 && i<=5
            v_line=vmax;
        elseif i>=6 && i<=10
            v_line=vmax-0.7;
        elseif i>=11 && i<=15
            v_line=vmax-1.4;
        elseif i>=16 && i<=20
            v_line=vmax-2.1;
        end
        V1(i,:) = -mysat(e1(i,:),vmax);
        if isnan(V1(i,1)) || isnan(V1(i,2))
            V1(i,:)=[0,0];
        end
        
        for j=1:N 
            if i~=j && any(Pcur(j,1:2)~=0)
                em = 0;
                ksimil = (Pcur(i,1:2) - Pcur(j,1:2)) ;
                bil = k2*dmysigma2(norm(ksimil),2*rs,rs+ra,em);
                V2(i,:) = V2(i,:)+ bil*(ksimil/norm(ksimil));
                if isnan(V2(i,1)) || isnan(V2(i,2))
                    V2(i,:)=[0,0];
                end
            end
        end
    
        et=0;
        ksii=Pcur(i,1:2);
        mksii=(A_mp*ksii'+b_mp)';
        rtksii=0.5*sqrt(ksii*(A_plpr'*A_plpr)*ksii'+ksii*A_plpr'*b_plpr+b_plpr'*A_plpr*ksii'+b_plpr'*b_plpr);
        ksiti = rtksii-norm(ksii - mksii);        
        dVtidksiti=k3*dmysigma2(ksiti,rs1(i),ra+rs1(i)-rs,et); 
        ci_direction=((drtpdp(ksii',A_plpr,b_plpr))'-((ksii - mksii)/norm(ksii - mksii))*(eye(2)-A_mp))';
        V3(i,:)=dVtidksiti*ci_direction';
        if isnan(V3(i,1)) || isnan(V3(i,2))
            V3(i,:)=[0,0];
        end
        
        if i~=j && any(Pcur(j,1:2)~=0)
            disti =  ksiti;
            dist_all(i)=ksiti;
            if disti<dist
                dist=disti;
            end
        end
        
    end

    V(i,:)=mysat(V1(i,:)+V2(i,:)+V3(i,:),vmax);

end

u=V;
ux = u(:,1);
uy = u(:,2);

== matlab function QuadrangleSimulation/MATLAB Function11 ==
  data: x input; Pcur output size=[N,2]
function Pcur  = fcn(x)
N=20;
Pcur=zeros(N,2);
for i=1:N
    Pcur(i,1)=x(i);
    Pcur(i,2)=x(i+N);
end
end
